simulink library "RxTxFixedPointLibrary_noscopes_mod"  (R2018a)
settings: Solver=VariableStepAuto  StartTime=0.0  StopTime=10.0  RelTol=1e-3
undefined symbols (not defined in the file): AGCBarkerSymbols, coeff, crcDecodeLag, CRCGeneratorLag, EQTrainingSymbols, j, K1, K2, numHeaderBits, numTrainingSamples, pLen, RadioSampleRate, samplesPerSymbol, VibertiTracebackLength, xPreambleSeq
libraries: simulink x33, dsphdlfiltering x20, hdlsllib x13, commseqgen3 x4, dspsigops x4, commdigbbndpm3 x3, commcrc2 x2, commcnvcod2 x2, RxTxFixedPointLibrary_noscopes x1, dspstat3 x1, commfilt2 x1
(part 3 of 3)

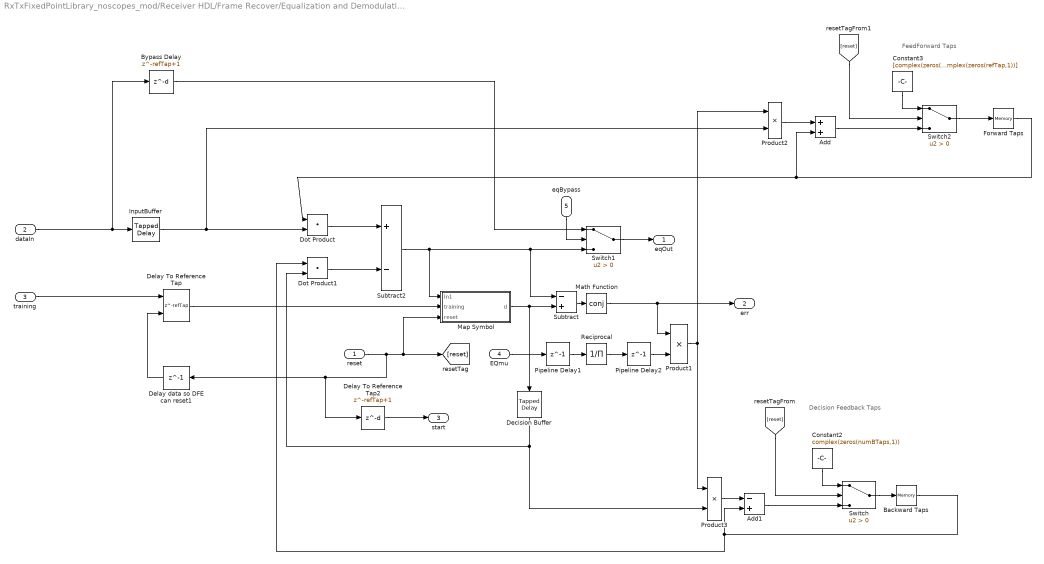
== system RxTxFixedPointLibrary_noscopes_mod/Receiver HDL/Frame Recover/Equalization and Demodulation/DFE/DFE ==
  note: Decision Feedback Taps
  note: FeedForward Taps
  reset : Inport
  dataIn : Inport  Port=2  OutDataTypeStr=fixdt(1,16,14)
  training : Inport  Port=3  OutDataTypeStr=fixdt(1,16,15)
  EQmu : Inport  Port=4
  eqBypass : Inport  Port=5
  Add : Sum  OutDataTypeStr=fixdt(1,16,14)
  Add1 : Sum  Inputs=-+  OutDataTypeStr=fixdt(1,16,19)
  Backward Taps : Memory  InitialCondition=complex(zeros(numBTaps,1))  InheritSampleTime=on
  Bypass Delay : Delay  DelayLength=refTap+1
  Constant2 : Constant  Value=complex(zeros(numBTaps,1))  OutDataTypeStr=fixdt(1,16,4)  SampleTime=-1
  Constant3 : Constant  Value=[complex(zeros(numFTaps-1-refTap,1));1;complex(zeros(refTap,1))]  OutDataTypeStr=fixdt(1,16,4)  SampleTime=-1
  Decision Buffer : simulink/Discrete/Tapped Delay  vinit=0.0  samptime=-1  NumDelays=numBTaps  DelayOrder=Oldest  includeCurrent=off
  Delay To Reference Tap : Delay  DelayLength=refTap  ExternalReset=Level
      settings: InputPortMap=u0,r5
  Delay To Reference Tap2 : Delay  DelayLength=refTap+1
  Delay data so DFE can reset1 : Delay  DelayLength=1
  Dot Product : DotProduct  OutDataTypeStr=fixdt(1,16,14)  SaturateOnIntegerOverflow=on  InputSameDT=on
  Dot Product1 : DotProduct  OutDataTypeStr=fixdt(1,16,18)  SaturateOnIntegerOverflow=on  InputSameDT=on
  Forward Taps : Memory  InitialCondition=[complex(zeros(numFTaps-1-refTap,1));1;complex(zeros(refTap,1))]  InheritSampleTime=on
  InputBuffer : simulink/Discrete/Tapped Delay  vinit=0.0  samptime=-1  NumDelays=numFTaps  DelayOrder=Oldest  includeCurrent=off
  Map Symbol : Subsystem
  Math Function : Math  Operator=conj  RndMeth=Zero  SaturateOnIntegerOverflow=on
  Pipeline Delay1 : Delay  DelayLength=1
  Pipeline Delay2 : Delay  DelayLength=1
  Product1 : Product  OutDataTypeStr=fixdt(1,16,22)
  Product2 : Product  OutDataTypeStr=fixdt(1,16,22)
  Product3 : Product  OutDataTypeStr=fixdt(1,16,21)
  Reciprocal : Product  Inputs=/  OutDataTypeStr=fixdt(0,16,22)  SaturateOnIntegerOverflow=on  RndMeth=Zero
  Subtract : Sum  Inputs=-+  OutDataTypeStr=fixdt(1,16,15)
  Subtract2 : Sum  Inputs=+-  OutDataTypeStr=fixdt(1,16,14)
  Switch : Switch  Criteria=u2 > Threshold  OutDataTypeStr=fixdt(1,16,15)
  Switch1 : Switch  Criteria=u2 > Threshold
  Switch2 : Switch  Criteria=u2 > Threshold  OutDataTypeStr=fixdt(1,16,14)
  eqOut : Outport
  err : Outport  Port=2
  start : Outport  Port=3
  wires:
  Math Function/1 -> Product1/1, err/1
  Product1/1 -> Product3/1, Product2/1
  EQmu/1 -> Pipeline Delay1/1
  Pipeline Delay2/1 -> Product1/2
  Pipeline Delay1/1 -> Reciprocal/1
  Reciprocal/1 -> Pipeline Delay2/1
  Delay To Reference Tap2/1 -> start/1
  Delay data so DFE can reset1/1 -> Delay To Reference Tap/2
  Delay To Reference Tap/1 -> Map Symbol/2(training)
  training/1 -> Delay To Reference Tap/1
  Product3/1 -> Add1/1
  Product2/1 -> Add/1
  [reset] -> Switch2/2
  Constant3/1 -> Switch2/1
  Add/1 -> Switch2/3
  Switch2/1 -> Forward Taps/1
  [reset] -> Switch/2
  Constant2/1 -> Switch/1
  Switch/1 -> Backward Taps/1
  Add1/1 -> Switch/3
  Decision Buffer/1 -> Dot Product1/2, Product3/2
  Backward Taps/1 -> Add1/2, Dot Product1/1
  reset/1 -> Map Symbol/3(reset), [reset], Delay data so DFE can reset1/1, Delay To Reference Tap2/1
  Map Symbol/1(d) -> Decision Buffer/1, Subtract/2
  Forward Taps/1 -> Add/2, Dot Product/1
  Subtract/1 -> Math Function/1
  Subtract2/1 -> Switch1/3, Subtract/1, Map Symbol/1(In1)
  Dot Product1/1 -> Subtract2/2
  Dot Product/1 -> Subtract2/1
  InputBuffer/1 -> Dot Product/2, Product2/2
  Switch1/1 -> eqOut/1
  dataIn/1 -> Bypass Delay/1, InputBuffer/1
  Bypass Delay/1 -> Switch1/1
  eqBypass/1 -> Switch1/2

== system RxTxFixedPointLibrary_noscopes_mod/Receiver HDL/Frame Recover/Equalization and Demodulation/DFE/Packeted To Unpacked ==
  In1 : Inport
  Extract Bits : simulink/Logic and Bit Operations/Extract Bits  bitsToExtract=Range of bits  numBits=8  bitIdxRange=[1]  outScalingMode=Treat bit field as an integer
      settings: SourceProductName=Simulink
  Extract Bits1 : simulink/Logic and Bit Operations/Extract Bits  bitsToExtract=Range of bits  numBits=8  bitIdxRange=[0]  outScalingMode=Treat bit field as an integer
      settings: SourceProductName=Simulink
  Vector Concatenate : Concatenate
  Out1 : Outport
  wires:
  Vector Concatenate/1 -> Out1/1
  Extract Bits1/1 -> Vector Concatenate/2
  Extract Bits/1 -> Vector Concatenate/1
  In1/1 -> Extract Bits/1, Extract Bits1/1

== system RxTxFixedPointLibrary_noscopes_mod/Receiver HDL/Frame Recover/Gardner Timing Recovery/Gardner TED Blocks/Imag Error ==
  data : Inport
  strobe sum : Inport  Port=2
  Delay : Delay  DelayLength=1
  Product1 : Product
  Sub : Sum  Inputs=+-
  TED Buffer Update1 : Subsystem
  Out1 : Outport
  wires:
  TED Buffer Update1/1(Middle Indx) -> Product1/1
  Delay/1 -> TED Buffer Update1/1(new data)
  TED Buffer Update1/2(oldest) -> Sub/1
  strobe sum/1 -> TED Buffer Update1/2(strobe sum)
  data/1 -> Delay/1, Sub/2
  Sub/1 -> Product1/2
  Product1/1 -> Out1/1

== system RxTxFixedPointLibrary_noscopes_mod/Receiver HDL/Frame Recover/Gardner Timing Recovery/Gardner TED Blocks/Real Error ==
  data : Inport
  strobe sum : Inport  Port=2
  Delay : Delay  DelayLength=1
  Product1 : Product  OutDataTypeStr=fixdt(1,16,12)
  Sub : Sum  Inputs=+-
  TED Buffer Update1 : Subsystem
  Out1 : Outport
  wires:
  TED Buffer Update1/1(Middle Indx) -> Product1/1
  Delay/1 -> TED Buffer Update1/1(new data)
  TED Buffer Update1/2(oldest) -> Sub/1
  strobe sum/1 -> TED Buffer Update1/2(strobe sum)
  data/1 -> Delay/1, Sub/2
  Sub/1 -> Product1/2
  Product1/1 -> Out1/1

== system RxTxFixedPointLibrary_noscopes_mod/Receiver HDL/Frame Recover/Gardner Timing Recovery/InterpControl_Blocks1/Calculate New mu ==
  note: Good at fixd(0,16,12)
  W : Inport
  NCOCounter : Inport  Port=2
  Math Reciprocal : Math  Operator=reciprocal  OutDataTypeStr=fixdt(1,16,12)  RndMeth=Zero  SaturateOnIntegerOverflow=on
  Product : Product  OutDataTypeStr=fixdt(0,15,14)
  mu : Outport
  wires:
  W/1 -> Math Reciprocal/1
  NCOCounter/1 -> Product/2
  Math Reciprocal/1 -> Product/1
  Product/1 -> mu/1

== system RxTxFixedPointLibrary_noscopes_mod/Receiver HDL/Frame Recover/Gardner Timing Recovery/InterpControl_Blocks1/Mod 1 ==
  In1 : Inport
  Add : Sum
  Compare To Constant : simulink/Logic and Bit Operations/Compare To Constant  relop=<  const=1  OutDataTypeStr=boolean
  Compare To Constant1 : simulink/Logic and Bit Operations/Compare To Constant  relop=>=  const=0  OutDataTypeStr=boolean
  Constant : Constant  OutDataTypeStr=fixdt(0,1,0)  SampleTime=-1
  Constant1 : Constant  OutDataTypeStr=fixdt(0,1,0)  SampleTime=-1
  Logical Operator : Logic  AllPortsSameDT=off  OutDataTypeStr=boolean
  Subtract : Sum  Inputs=+-
  Switch : Switch  Criteria=u2 > Threshold
  Switch1 : Switch
  Out1 : Outport
  wires:
  Logical Operator/1 -> Switch/2
  Compare To Constant/1 -> Logical Operator/2
  Compare To Constant1/1 -> Logical Operator/1
  In1/1 -> Subtract/1, Add/1, Switch/1, Compare To Constant/1, Compare To Constant1/1, Switch1/2
  Add/1 -> Switch1/3
  Subtract/1 -> Switch1/1
  Switch1/1 -> Switch/3
  Constant1/1 -> Add/2
  Constant/1 -> Subtract/2
  Switch/1 -> Out1/1

== system RxTxFixedPointLibrary_noscopes_mod/Transmitter HDL/Packet Generation/Payload/HDL Scrambler/Resettable Synchronous Subsystem ==
  In1 : Inport
  Reset : ResetPort  DisableCoverage=on  ResetTriggerType=level hold
  Delay2 : Delay  DelayLength=1  InitialCondition=false
  State Control : StateControl  StateControl=Synchronous
  Tapped Delay : simulink/Discrete/Tapped Delay  vinit=init_state(1:end-1)  samptime=-1  NumDelays=length(init_state)-1  DelayOrder=Oldest  includeCurrent=on
  Out1 : Outport
  wires:
  Tapped Delay/1 -> Out1/1
  In1/1 -> Delay2/1
  Delay2/1 -> Tapped Delay/1

== system RxTxFixedPointLibrary_noscopes_mod/Receiver HDL/Frame Recover/Equalization and Demodulation/DFE/DFE/Map Symbol ==
  In1 : Inport  OutDataTypeStr=fixdt(1,16,14)
  training : Inport  Port=2  OutDataTypeStr=fixdt(1,16,15)
  reset : Inport  Port=3
  Decision Directed : Subsystem
  Delay : Delay  DelayLength=1
  HDL Counter : hdlsllib/Sources/HDL Counter  CountType=Count limited  CountInit=0  CountStep=1  CountMax=2^18  CountFromType=Initial value  CountFrom=0  CountResetPort=on  CountLoadPort=off  CountEnbPort=off  CountDirPort=off  CountDataType=Unsigned  CountWordLen=32  CountFracLen=0  CountSampTime=1
      settings: SourceProductBaseCode=HD
  Switch : Switch  Criteria=u2 > Threshold  Threshold=numTrainingSamples  OutDataTypeStr=fixdt(1,16,15)
  d : Outport
  wires:
  Delay/1 -> Switch/3
  training/1 -> Delay/1
  Decision Directed/1(decision) -> Switch/1
  HDL Counter/1 -> Switch/2
  reset/1 -> HDL Counter/1
  Switch/1 -> d/1
  In1/1 -> Decision Directed/1(eqOut)

== system RxTxFixedPointLibrary_noscopes_mod/Receiver HDL/Frame Recover/Gardner Timing Recovery/Gardner TED Blocks/Imag Error/TED Buffer Update1 ==
  new data : Inport
  strobe sum : Inport  Port=2
  Delay{,1..3} (4 alike) : Delay  DelayLength=1
  Multiport Switch{,1..3} (4 alike) : MultiPortSwitch  DataPortOrder=Zero-based contiguous  DataPortIndices={0,1,[2,3]}  zeroidx=on
  Zero bit : Constant  Value=0  OutDataTypeStr=fixdt(1,16,13)  SampleTime=1/RadioSampleRate
  Middle Indx : Outport
  oldest : Outport  Port=2
  wires:
  Multiport Switch/1 -> oldest/1, Delay/1
  Multiport Switch3/1 -> Delay3/1
  Multiport Switch2/1 -> Delay2/1, Middle Indx/1
  Multiport Switch1/1 -> Delay1/1
  Delay3/1 -> Multiport Switch3/2, Multiport Switch2/3, Multiport Switch1/4
  Zero bit/1 -> Multiport Switch2/4
  new data/1 -> Multiport Switch3/3, Multiport Switch3/4
  Delay2/1 -> Multiport Switch2/2, Multiport Switch1/3, Multiport Switch/4
  Delay1/1 -> Multiport Switch1/2, Multiport Switch/3
  Delay/1 -> Multiport Switch/2
  strobe sum/1 -> Multiport Switch/1, Multiport Switch1/1, Multiport Switch2/1, Multiport Switch3/1

== system RxTxFixedPointLibrary_noscopes_mod/Receiver HDL/Frame Recover/Gardner Timing Recovery/Gardner TED Blocks/Real Error/TED Buffer Update1 ==
  new data : Inport
  strobe sum : Inport  Port=2
  Delay{,1..3} (4 alike) : Delay  DelayLength=1
  Multiport Switch{,1..3} (4 alike) : MultiPortSwitch  DataPortOrder=Zero-based contiguous  DataPortIndices={0,1,[2,3]}  zeroidx=on
  Zero bit : Constant  Value=0  OutDataTypeStr=fixdt(1,16,13)  SampleTime=1/RadioSampleRate
  Middle Indx : Outport
  oldest : Outport  Port=2
  wires:
  Multiport Switch/1 -> oldest/1, Delay/1
  Multiport Switch3/1 -> Delay3/1
  Multiport Switch2/1 -> Delay2/1, Middle Indx/1
  Multiport Switch1/1 -> Delay1/1
  Delay3/1 -> Multiport Switch3/2, Multiport Switch2/3, Multiport Switch1/4
  Zero bit/1 -> Multiport Switch2/4
  new data/1 -> Multiport Switch3/3, Multiport Switch3/4
  Delay2/1 -> Multiport Switch2/2, Multiport Switch1/3, Multiport Switch/4
  Delay1/1 -> Multiport Switch1/2, Multiport Switch/3
  Delay/1 -> Multiport Switch/2
  strobe sum/1 -> Multiport Switch/1, Multiport Switch1/1, Multiport Switch2/1, Multiport Switch3/1

== system RxTxFixedPointLibrary_noscopes_mod/Receiver HDL/Frame Recover/Equalization and Demodulation/DFE/DFE/Map Symbol/Decision Directed ==
  eqOut : Inport  OutDataTypeStr=fixdt(1,16,14)
  Compare To Zero : simulink/Logic and Bit Operations/Compare To Zero  relop=>=  OutDataTypeStr=boolean
  Compare To Zero1 : simulink/Logic and Bit Operations/Compare To Zero  relop=>=  OutDataTypeStr=boolean
  Complex to Real-Imag : ComplexToRealImag
  QPSK Decisions : LookupNDDirect  Table=[-0.7071 - 0.7071i, -0.7071 + 0.7071i; 0.7071 - 0.7071i, 0.7071 + 0.7071i]  DiagnosticForOutOfRangeInput=Error  TableDataTypeStr=fixdt(1,16,15)
  decision : Outport
  wires:
  QPSK Decisions/1 -> decision/1
  Compare To Zero1/1 -> QPSK Decisions/2
  Compare To Zero/1 -> QPSK Decisions/1
  Complex to Real-Imag/2 -> Compare To Zero1/1
  Complex to Real-Imag/1 -> Compare To Zero/1
  eqOut/1 -> Complex to Real-Imag/1

== matlab function RxTxFixedPointLibrary_noscopes_mod/Receiver HDL/Frame Recover/Frequency Recovery/Lock Detector/MATLAB Function ==
  data: u input; y output
function y = abs(u)

y = fi(u,0,16,10);

== matlab function RxTxFixedPointLibrary_noscopes_mod/Transmitter HDL/Packet Generation/Payload/Viterbi Lag Stuffer/MATLAB Function ==
  data: enable input; reset output; mode output
function [reset,mode] = fcn(enable)

persistent counter

if isempty(counter)
   counter = uint8(0);
end

if enable
    counter = uint8(34*2); % tracebacklength*2
    mode = uint8(1);
    reset = true;
elseif counter>uint8(0)
    counter = counter - 1;
    mode = uint8(1);
    reset = false;
else
    mode = uint8(0);
    reset = false;
end

== matlab function RxTxFixedPointLibrary_noscopes_mod/Receiver HDL/Frame Recover/Gardner Timing Recovery/TED Lock Detector/MATLAB Function ==
  data: u input; y output
function y = abs(u)

y = fi(u,0,16,15);

== matlab function RxTxFixedPointLibrary_noscopes_mod/Receiver HDL/Viterbi Decode/Descrambler1/MATLAB Function ==
  data: data input; vec output; reset input
function vec = ResetableTapDelay(data,reset)

persistent buffer

if isempty(buffer)
    buffer = [0 1 0 0 0 1 0]>0;
end
    
if reset
    vec = [0 1 0 0 0 1 0]>0;
    buffer = [0 1 0 0 0 1 0]>0;
else
   vec = [buffer(2:end),data];
   buffer = [buffer(2:end),data];
end

== matlab function RxTxFixedPointLibrary_noscopes_mod/Transmitter HDL/Packet Generation/Payload/Latch/MATLAB Function3 ==
  data: start input; enable output; done input
function enable = latch(start,done)

persistent state

if isempty(state)
   state = false; 
end

if start
    enable = true;
    state = true;
elseif done
    enable = true;
    state = false;
else
    enable = state;
end

== matlab function RxTxFixedPointLibrary_noscopes_mod/Receiver HDL/CRC Check and DMA Pack/DMA Interface/Bit Packer ==
  data: bitIn input; byteOut output; startIn input; endIn input; err input; validIn input; validOut output; startOut output; endOut output
function [byteOut,validOut,startOut,endOut] = BitPacker(bitIn, startIn, endIn, err, validIn)

% This block will pack bits into bytes with start boundaries


% Constants
bits2Pack = uint8(64); % byteReg must contain this many bits
zero64 = fi(0,0,64,0);
% NOTE: Frames but be a multiple of bits2Pack or bits will be trimmed from
% end

persistent byteReg byteIndx setStartFlag

if isempty(byteIndx)
    byteReg  = fi(0,0,64,0);
    byteIndx = uint8(1);
    setStartFlag = false;
end

if validIn
    if startIn % Reset
        byteReg = bitset(zero64,1,bitIn);
        byteIndx = uint8(2);
        validOut = false;
        setStartFlag = true;
        startOut = false;
    else
        byteReg = bitset(byteReg,byteIndx,bitIn);
        if byteIndx >= bits2Pack
            byteIndx = uint8(1);
            validOut = true;
            startOut = setStartFlag;
            setStartFlag = false;
        else
            byteIndx = byteIndx + uint8(1);
            validOut = false;
            startOut = false;
        end
    end
    endOut = false;
elseif endIn % Append error bit to last byte
    byteReg = fi(err,0,64,0);
    validOut = true;
    startOut = false;
    endOut = true;
else
    validOut = false;
    startOut = false;
    endOut = false;
end

byteOut = byteReg;

== matlab function RxTxFixedPointLibrary_noscopes_mod/Receiver HDL/Frame Recover/Enable Equalizer and Packet Decode (Latch) ==
  data: start input; enable output; validIn input
function enable = Counter(start,validIn)

persistent count maxCount lastEOF

if isempty(count)
    count = uint32(0);
    maxCount = uint32(2^16); % Largest possible packet length
    lastEOF = false;
end

eof = false;

if validIn
    % Got a barker preamble start allowing data into equalizer
    if start
        count = maxCount;
    end
    
    % Check on change from true to false
    if lastEOF && ~eof
        %     fprintf('Frame end reached\n');
        count = uint32(0);
    end
    lastEOF = eof;
    
    % Past end of max frame size
    if count>0
        count = count - uint32(1);
    end
    
    % Enable downstream
    enable = count>uint32(0);
else
    enable = false;
end

== matlab function RxTxFixedPointLibrary_noscopes_mod/Receiver HDL/Frame Recover/Manage Error Signals/Debug: Header Check/DEBUG: Header ==
  data: status input; h1 input; h2 input
function HeaderDebug(status,h1,h2)

if status==uint8(2)
    fprintf('Header Check failed (possible false detection)\n');
    fprintf('sum1: %d\n',int32(h1));
    fprintf('sum2: %d\n',int32(h2));
elseif status==uint8(1)
    fprintf('Header Found | Packet is %d bits long\n',int32(h1));
end

== matlab function RxTxFixedPointLibrary_noscopes_mod/Receiver HDL/Frame Recover/Equalization and Demodulation/DFE/Equalizer ==
  data: trigger input; eqOut output; data input; trainingSymbol input
function eqOut  = dfe(trigger,data,trainingSymbol)

persistent inputBuffer decisionBuffer forwardTaps backwardTaps processedSamples


%% Constants
WL = uint8(16); FL = uint8(14);
F = fimath('SumMode','SpecifyPrecision','SumWordLength',WL,...
    'SumFractionLength',FL);
% Initial delay guess
channelDelay = uint8(0);
% Equalizer settings
mu = fi(0.05,0,10,12);
nFTaps = uint8(11);
nBTaps = uint8(3);
numTrainingSymbols = uint16(250);
resetTaps = fi([complex(zeros(nFTaps-1,1));1],1,WL,FL,F);

%% Async
if isempty(inputBuffer)
    % Set Precisions
    inputBuffer = fi(complex(zeros(nFTaps,1)),1,WL,FL,F);
    decisionBuffer = fi(complex(zeros(nBTaps,1)),1,WL,FL,F);
    forwardTaps = fi(complex(zeros(nFTaps,1)),1,WL,FL,F);
    backwardTaps = fi(complex(zeros(nBTaps,1)),1,WL,FL,F);
    processedSamples = numTrainingSymbols + uint16(1); % Force to DD mode to start
end

%% Reset
if trigger
    processedSamples = uint16(0);
    % Reset taps
    %forwardTaps = fi(complex(zeros(nFTaps,1)),1,WL,FL,F);
    %forwardTaps(nFTaps-channelDelay) = fi(1,1,WL,FL); % Favor specific delay (causes equalizer to converge faster)
    forwardTaps = resetTaps;
    backwardTaps = fi(complex(zeros(nBTaps,1)),1,WL,FL,F);
    % Default output
    eqOut = fi(0,1,WL,FL,F);
else
    %% Equalizer
    % Add data to buffer
    inputBuffer = [inputBuffer(2:end);data];
    
    % Apply equalizer
    eqOut = forwardTaps'*inputBuffer - backwardTaps'*decisionBuffer;
    
    % Determine error
    if (processedSamples<numTrainingSymbols) && (processedSamples>=channelDelay)
        processedSamples = processedSamples + 1;
        d = trainingSymbol;
    else % Decision directed
        % Find closest symbol
        r = real(eqOut)>0; i = imag(eqOut)>0;
        if r
            if i
                d = fi(0.7071 + 0.7071i,1,WL,FL);
            else
                d = fi(0.7071 - 0.7071i,1,WL,FL);
            end
        else
            if i
                d = fi(-0.7071 + 0.7071i,1,WL,FL);
            else
                d = fi(-0.7071 - 0.7071i,1,WL,FL);
            end
        end
    end
    ec = conj(d - eqOut);
    
    % Update taps
    forwardTaps = forwardTaps + mu*ec*inputBuffer;
    backwardTaps = backwardTaps - mu*ec*decisionBuffer;
    
    % Update decision buffer
    db = fi(d,1,WL,FL,F);
    decisionBuffer = [db; decisionBuffer(1:end-1)];
    
end



end

== matlab function RxTxFixedPointLibrary_noscopes_mod/Receiver HDL/Frame Recover/Equalization and Demodulation/Header Controller ==
  data: enableDownstream output; headerStart input; packetLenBitsOut output; data input; resetViterbi output; crcStart output; status output; s1 output; s2 output
function [enableDownstream,packetLenBitsOut,resetViterbi,crcStart,status,s1,s2] = EvalHeader(headerStart, data)

persistent counter sum1 sum2 packetLenBits lastMode savedPacketLenBits

% The header contains 16 bits, but each bit is duplicated to make checking
% easier
%
% Note this block works on symbols (2bits) but 1 symbol -> 1 decoded bit
%
% PacketLength = (Data+CRC+40(TB)+68)/CodeRate
%
% NOTE TAIL BITS HERE ARE REALLY USED TO DEAL WITH VITERBI LAG SO:
% TailBitsWithLagPadding > TracebackLength

%% Constants
numHeaderBits = uint8(16); % Header is this many bits
powersOfTwo = uint32([1 2 4 8 16 32 64 128 256 512 1024 2048 4096 8192 16384 32768]);
CodeRateINV = uint32(2);%1/CodeRate;
TailBitsWithLagPadding = uint32(uint32(40)+34*2+1); % was +1
% Flag when CRC porition of packet starts relative to header
crcSignalStartLocation = uint32(0);%uint32((TailBitsWithLagPadding)*CodeRateINV); % Must be even

% Async
if isempty(counter)
    packetLenBits = uint32(0);
    sum1 = uint32(0);
    sum2 = uint32(0);
    counter = uint8(numHeaderBits);
    lastMode = uint8(3);
    savedPacketLenBits = uint16(0);
end


%% Sync
% Got a header now enable certain mode
if headerStart && (lastMode==3)
    mode = uint8(0);
else
    mode = lastMode;
end

switch mode
    %% Reset on preamble flag and setup for header processing
    case uint8(0)
        crcStart = false;
        resetViterbi = false;
        enableDownstream = false;
        sum1 = uint32(0);
        sum2 = uint32(0);
        counter = uint8(1);
        lastMode = uint8(1); % Go to next state
        packetLenBitsOut = uint16(0);
        status = uint8(0); s1 = uint32(0); s2 = uint32(0);
        
    %% Process header
    case 1 
        crcStart = false;
        enableDownstream = false;
        
        % Convert header bits (bit by bit)
        if data(1)
            sum1 = sum1 + powersOfTwo(counter);
        end
        if ~data(2)
            sum2 = sum2 + powersOfTwo(counter);
        end
        counter = counter + uint8(1);
        
        if counter>numHeaderBits
            % Check header
            if (sum1~=sum2) || (sum1==0) % Fail
                packetLenBits = uint32(0);
                lastMode = uint8(3);
                resetViterbi = false;
                packetLenBitsOut = uint16(0);
                savedPacketLenBits = uint16(0);
                status = uint8(2); s1 = sum1; s2 = sum2;
            else % Pass
                % Saved header info and trigger downstream
                packetLenBits = uint32(sum1);
                lastMode = uint8(2);
                resetViterbi = true;
                packetLenBitsOut = uint16(sum1-crcSignalStartLocation);
                savedPacketLenBits = uint16(sum1-crcSignalStartLocation);
                status = uint8(1); s1 = sum1; s2 = sum2;
            end
        else
            status = uint8(0); s1 = uint32(0); s2 = uint32(0);
            packetLenBitsOut = uint16(0);
            resetViterbi = false;
        end
        
    %% Decrement sample counter
    case 2 
        status = uint8(0); s1 = uint32(0); s2 = uint32(0);
        resetViterbi = false;
        crcStart = (packetLenBits==crcSignalStartLocation);
        if packetLenBits>uint32(0)
            enableDownstream = true;
            packetLenBits = packetLenBits - uint32(2); % We get 2 bits each call
            packetLenBitsOut = savedPacketLenBits;
        else
            enableDownstream = false;
            lastMode = uint8(3);
            packetLenBitsOut = uint16(0); %Reset
            savedPacketLenBits = uint16(0);%Reset
        end
            
    %% Not processing anything
    otherwise % mode>2
        status = uint8(0); s1 = uint32(0); s2 = uint32(0);
        crcStart = false;
        resetViterbi = false;
        enableDownstream = false;
        packetLenBitsOut = uint16(0);
end

== matlab function RxTxFixedPointLibrary_noscopes_mod/Receiver HDL/Frame Recover/Frequency Recovery/PED ==
  data: In input; e output
function e  = PED(In)

OP2 = real(In);
OP1 = imag(In);

Real = OP2;
Imag = OP1;

if (bitget(Real,16)==true) % real component is negative
    OP1 = fi(-Imag,1,16,13);
end
if (bitget(Imag,16)==true) % imaginary component is negative
    OP2 = fi(-Real,1,16,13);
end

e= fi(OP1-OP2,1,16,10);

%e = sign(real(In)).*imag(In) - sign(imag(In)).*real(In);

== matlab function RxTxFixedPointLibrary_noscopes_mod/Transmitter HDL/DMA Interface/DMA Control ==
  data: byteIn input; validIn input; EOF input; modeIn input; bitOut output; validOut output; startOut output; payloadLength output; readyForInput output; modeOut output; bitCounterIn input; bitCounterOut output; inputByteCounterIn input; inputByteCounterOut output
function [bitOut,validOut,startOut,payloadLength,readyForInput,modeOut,bitCounterOut,inputByteCounterOut] = DMA_Control(byteIn,validIn,EOF,modeIn,bitCounterIn,inputByteCounterIn)

% This block converts the byte input pipeline into bits and extract the
% length the packet into its own signal

persistent wordBuffer payloadLenBuff gapCounter

bitsInInput = uint8(64);
bytesInInput = uint16(8);
gapBetweenValids = uint8(8);

if isempty(wordBuffer)
    wordBuffer = fi(0,0,64,0); % Must match number of bits defined by bitsInInput
    payloadLenBuff = uint16(0);
    gapCounter = uint8(0);
end


switch modeIn
    %% Startup and wait
    case uint8(0)
        if validIn
            % At this state the word received will be the payload length
            % which is used by downstream blocks to construct header
            modeOut = uint8(5);
            payloadLenBuff = uint16(byteIn);
            % Set outputs
            bitOut = false;
            validOut = false;
            startOut = false;
            payloadLength = uint16(0);
            readyForInput = true; % Request next word
            % Reset counters
            inputByteCounterOut = bytesInInput;% Reset
            bitCounterOut = uint8(1);% Reset
        else
            % Set main outputs
            bitOut = false;
            if modeIn == uint8(0)
                validOut = true; % Let LFSR Run
            else
                validOut = false;
            end
            startOut = false;
            payloadLength = uint16(0);
            modeOut = uint8(modeIn);
            bitCounterOut = uint8(1);
            inputByteCounterOut = bytesInInput;
            % Determine DMA call
            if modeIn == uint8(2)
                readyForInput = false;
            else
                % New payload words should only come every 4 cycles
                if gapCounter>=gapBetweenValids
                    gapCounter = uint8(1);
                    readyForInput = true;
                else
                    gapCounter = gapCounter + uint8(1);
                    readyForInput = false;
                end            
            end
        end
    %% Wait for delay of valid
    case uint8(5)
        bitCounterOut = uint8(2);
        if validIn % Got next word
            modeOut = uint8(2);
            bitOut = bitget(byteIn,1)>0;
            wordBuffer = byteIn; % Save byte
            validOut = true;
            startOut = true;
            readyForInput = true;
        else
            modeOut = uint8(5);
            bitOut = false;
            validOut = false;
            startOut = false;
            readyForInput = false;
        end
        % Set outputs
        payloadLength = uint16(0);
        % Reset counters
        inputByteCounterOut = inputByteCounterIn;% Reset
        
    %% Payload output
    case uint8(2)
        % Output each word 1 bit at a time
        if bitCounterIn==uint8(1)
            bitOut = bitget(byteIn,1)>0;
            wordBuffer = byteIn; % Save byte
            readyForInput = inputByteCounterIn<payloadLenBuff; % Queue up next word
        else
            bitOut = bitget(wordBuffer,bitCounterIn)>0;
            readyForInput = false;
        end
        payloadLength = uint16(payloadLenBuff);
        validOut = true && (inputByteCounterIn >= bytesInInput); % SKIP FIRST WORD 
        startOut = false;
        % Set flag to DMA and next mode
        if bitCounterIn >= uint8(bitsInInput)
            bitCounterOut = uint8(1); % Reset
            % If we've processed all the bytes we need to wait for downstream
            % to be done
            if inputByteCounterIn<payloadLenBuff
                modeOut = uint8(2); % 
                % Bytes processed
                inputByteCounterOut = inputByteCounterIn + bytesInInput;
            else
                %readyForInput = false; % Hold DMA off for now, next call will go to EOF
                modeOut = uint8(3);
                inputByteCounterOut = uint16(inputByteCounterIn);
                %startOut = false;
            end
        else
            modeOut = uint8(2);
            bitCounterOut = bitCounterIn+uint8(1);
            inputByteCounterOut = uint16(inputByteCounterIn);
        end
        
    %% Waiting for EOF from packet generation
    otherwise %case uint8(3)
        bitOut = false;
        validOut = true; % Keep downstream processing going
        startOut = false;
        payloadLength = uint16(payloadLenBuff);
        if EOF % Done with frame now ask for more data
            %readyForInput = true;
            readyForInput = false;
            modeOut = uint8(0);% Reset
        else
            readyForInput = false;
            modeOut = uint8(3);
        end
        % Not used
        bitCounterOut = uint8(1);
        inputByteCounterOut = bytesInInput;
        
end

== matlab function RxTxFixedPointLibrary_noscopes_mod/Transmitter HDL/Packet Generation/Tx Controller ==
  data: modeOut output; headerData output; data output; payloadBit input; payloadSize input; count input; start input; dataStart output; dataEnd output; preambleReset output
function [modeOut, headerData, data, dataStart, dataEnd, preambleReset] = fcn(payloadBit,payloadSize,count, start)

% When we get a start flag buffers are reset and the next cycle with start
% in mode 0

% Reset: New payload size is passed at an int16
% 


persistent  headerBits numPayloadBits mode

numHeaderBits = uint32(16);
AGCBarkerSymbols = 160+28;
EQTrainingSymbols = 250; % 2 bits per symbol => 250 symbols
preambleBits = uint32(EQTrainingSymbols+AGCBarkerSymbols-0);
CRCLength = 32;
CRCGeneratorLag = CRCLength+2+0; % additional 1 is from reset of encoder
CodeRate = 2;
lagBits = 40+68;
viterbiTraceback = uint32(34*2);

% Async/Init
if isempty(numPayloadBits)
    % Sizes of frame sections
    numPayloadBits = uint32(0); 
    %headerBits = zeros(1,numHeaderBits)>0;
    headerBits = uint16(0);
    mode = uint8(4);
end

% Synchronous
switch mode
    case uint8(0) % Reset
        % Move to next mode on next input/clock
        mode = uint8(1);
        % Convert payloadSize to bits
        numPayloadBits = uint32(bitshift(payloadSize,3)+CRCLength);
        %headerBits = logical(bitget(CodeRate*(payloadSize+CRCLength),1:numHeaderBits));
        headerBits = uint16(bitshift((bitshift(payloadSize,3)+CRCLength+lagBits),1));        
        % Set outputs
        modeOut = uint8(4);
        headerData = false;
        data = false; % Not used downstream
        dataStart = false;
        dataEnd = false;
        preambleReset = true;
    case uint8(1) % Preamble
        % Set Next Mode
        if count>=(preambleBits)
            preambleReset = false;
            mode = uint8(2);
        elseif count==uint32(1)
            preambleReset = false;
            mode = uint8(1);
        else
            preambleReset = false;
            mode = uint8(1);
        end
        % Set outputs
        modeOut = uint8(1);
        headerData = false;
        % Start outputing data early to compensate for CRC lag
        if count>=(preambleBits+numHeaderBits-CRCGeneratorLag)
           data = payloadBit;
        else
           data = false;         
        end
        % Set flag on first payload bit
        dataStart = count == (preambleBits+numHeaderBits-CRCGeneratorLag-uint32(1)); % This will occur 1 cycle early to reset scrambler
        % Cannot reach data yet
        dataEnd = false;
    case uint8(2) % Header bits
        % Set Next Mode
        if count>=(preambleBits+numHeaderBits)
            mode = uint8(3);
        else
            mode = uint8(2);
        end
        % Set outputs
        modeOut = uint8(2);
        %headerData = headerBits(count-preambleBits);
        headerData = bitget(headerBits,count-preambleBits)>0;
        data = payloadBit;
        dataStart = false;
        dataEnd = false;
        preambleReset = false;
    case uint8(3) % Payload bits and CRC
        % Set Next Mode
        if count>=(preambleBits+numHeaderBits+numPayloadBits+viterbiTraceback)%+CRCGeneratorLag)
            % Will coencide with last CRC Bit (NOT TRUE ANYMORE WILL BE ON
            % LAST TRACEBACK PADDING BIT)
            mode = uint8(4);
        else
            mode = uint8(3);
        end
        % Set outputs
        modeOut = uint8(3);        
        headerData = false;
        data = payloadBit;
        % Set flag on last payload bit
        dataStart = false;
        dataEnd =   ( count==(preambleBits+numHeaderBits+numPayloadBits-CRCLength-CRCGeneratorLag-1) );
        preambleReset = false;
    otherwise %case uint8(4) % Waiting for data
        % Chilling for new start
        if start
           mode = uint8(0); 
        else
           mode = uint8(4);
        end
        % Set outputs
        modeOut = uint8(4);
        headerData = false;
        data = false; % Not used downstream
        dataStart = false;
        dataEnd = false;
        preambleReset = false;
end
